simulink model "filecuaho"  (R2016b)
settings: Solver=VariableStepAuto  StartTime=0.0  StopTime=10.0  RelTol=1e-3
undefined symbols (not defined in the file): KACC_ACCT_CLR_NIDL_INIT, KACC_ACCUT_STATE_A, KACC_ACCUT_STATE_B, KACC_ACCUT_SW, KACC_ACTQSW, KACC_CLD, KACC_CLD_REQ_HYS, KACC_CLD_REQ_SW, KACC_COLPD, KACC_COMP_INRT, KACC_COMPTYPE_FIXED, KACC_COMPTYPE_VAR, KACC_CTTM_ACE, KACC_CTTM_ACON, KACC_CTTM_CRK, KACC_CTTM_FAN, KACC_CTTM_GRD, KACC_CTTM_IRS, KACC_CTTM_NAC, KACC_DIFFEVATEMPMAX, KACC_DIFFEVATEMPMIN, KACC_EVAT_ELSE, KACC_EVAT_ELSE_SW, KACC_EVATMPCUT_SW, KACC_EVATUPL_ELSE, KACC_EVATUPL_ELSE_SW, KACC_FANREQ_SW, KACC_FORCEDACON, KACC_HCAPS, KACC_HCAPS_HYS, KACC_HCCTTM, KACC_HCGRA, KACC_HCGRA_HYS, KACC_HCRGR, KACC_HCVS1, KACC_HCVS1_HYS, KACC_HCVS2, KACC_HCVS2_HYS, KACC_HEATUP_CE, KACC_HEATUP_CE_HYS, KACC_HEATUP_DRV2IDL, KACC_HEATUP_IDL2DRV, KACC_HEATUP_NE, KACC_HEATUP_NE_HYS, KACC_HIPS_ACOF, KACC_HIPS_ACON, KACC_LOPS_ACOF, KACC_LOPS_ACON, KACC_LYR3TR_ACHLD, KACC_NEW_RPM, KACC_OFDL_SW, KACC_OFDL_VCV, KACC_ONDL_SW, KACC_RECCP, KACC_RECCP_HYS, KACC_RECDLY, KACC_RECVS, KACC_S1_THWMAX, KACC_S1TM_THWULMT, KACC_SHLT_2CYL ... (+137)
libraries: lib2011b x727, SUBSYSTEM_LIB_CNV x30, SUBSYSTEM_LIB_ESC x2, SUBSYSTEM_LIB_AUX x1
(part 3 of 5)

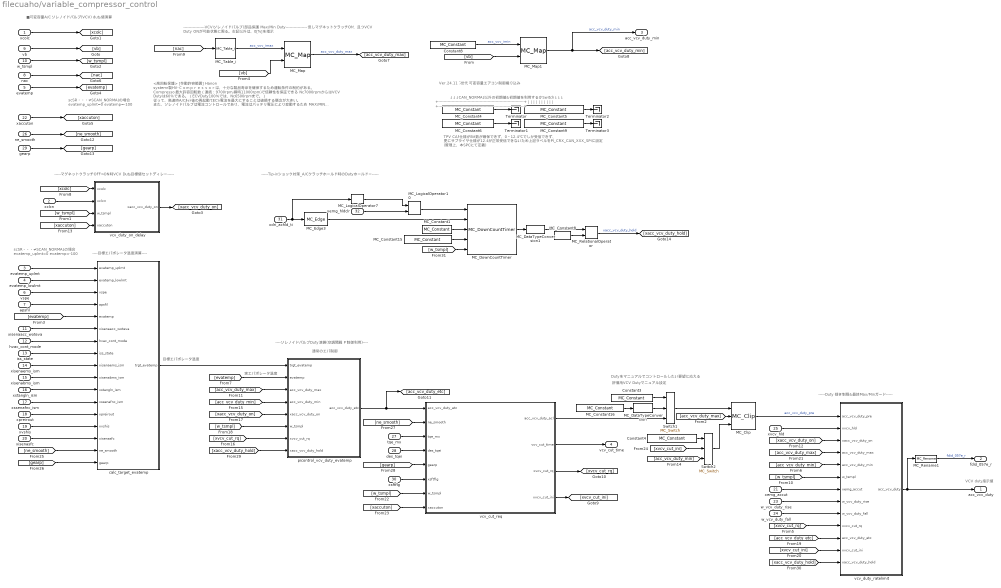
== system filecuaho/variable_compressor_control ==
  note: ■可変容量A/C ソレノイドバルブ(VCV) duty値演算
  note: VCV duty指示値
  note: <高回転保護>
      | [作動許容範囲]
      | Hanon systems製HV-Ｃｏｍｐｒｅｓｓｏｒは、十分な製品寿命を確保するため運転条件の制約がある。
      | Compressor最大許容回転数（連続：9700rpm/瞬時11000rpm)で信頼性を保証できる
      | Nc7000rpmからはVCV Dutyは60％である。（ECVDuty100％では、Nc6500rpmまで。）
      | 従って、高速時A/Cｶｯﾄ後の再起動でECV電流を最大にすることは破損する懸念が大きい。
      | また、ソレノイドバルブは電流コントロールであり、電流はバッテリ電圧により変動するため
      | MAX/MIN Dutyは電圧補正を行う
  note: 評価用VCV Dutyマニュアル設定
  note: Dutyをマニュアルでコントロールしたい要望に応える
  note: 通常のエバ制御
  note: 目標エバポレータ温度
  note: 実エバポレータ温度
  note: ----ソレノイドバルブDuty演算(空調開殿 PI制御利用)----
  note: scSR・・・≠SCAN_NORMALの場合
      |  evatemp_uplmt=0
      |  evatemp=-100
  note: ----目標エバポレータ温度演算----
  note: ----------------VCV(ソレノイドバルブ)部品保護 Max/Min Duty----------------
      | 但しマグネットクラッチON、且つVCV Duty ONが可能状態に限る。左記以外は、0[%]を指示
  note: scSR・・・≠SCAN_NORMALの場合
      |  evatemp_uplmt=0
      |  evatemp=-100
  note: -----マグネットクラッチOFF⇒ON時VCV Duty目標値セットディレー-----
  note: -----Duty 傾き制限&最終Max/Minガード-----
  note: ↓↓↓CAN_NORMAL以外の初期値&初期値を利用するかSwitch↓↓↓
  note: TPV CAN仕様がBit数が確保できず、0～12.4℃でしか受信できず、
      | 更にサプライヤ仕様が12.4が正常受信できないため上記ラベルをPI_CRX_CAN_XXX_SPCに設定
      | (管理上、本SPCにて定義)
  note: +----------------------------------------------------------------+
      | |                                                                                                                            　   |
      | |                                                                                                                            　   |
      | |                                                                                                                            　   |
      | |                                                                                                                            　   |
      | |                                                                                                                            　   |
      | +----------------------------------------------------------------+
  note: Ver.24.11
      | 7世代 可変容量エアコン制御織り込み
  note: -----Tip-inショック対策_A/Cクラッチホールド時のDutyホールドー-----
  xcolc : Inport
  xclcn : Inport  Port=2
  evatemp_uplmt : Inport  Port=3
  evatemp_lowlmt : Inport  Port=4
  evatemp : Inport  Port=5
  vspe : Inport  Port=6
  apsfil : Inport  Port=7
  nac : Inport  Port=8
  vb : Inport  Port=9
  w_tsmpl : Inport  Port=10
  xisenaacc_woteva : Inport  Port=11
  hvac_cont_mode : Inport  Port=12
  iss_state : Inport  Port=13
  xisenaems_ism : Inport  Port=14
  xisenabms_ism : Inport  Port=15
  xstangln_ism : Inport  Port=16
  xssenafnc_ism : Inport  Port=17
  xpreirout : Inport  Port=18
  xvshis : Inport  Port=19
  xisenasfc : Inport  Port=20
  xemg_accut : Inport  Port=21
  xaccuton : Inport  Port=22
  w_vcv_duty_rise : Inport  Port=23
  w_vcv_duty_fall : Inport  Port=24
  xvcv_hld : Inport  Port=25
  ne_smooth : Inport  Port=26
  tqe_mx : Inport  Port=27
  des_tqei : Inport  Port=28
  gearp : Inport  Port=29
  xsftflg : Inport  Port=30
  xdri_achld_ti : Inport  Port=31
  xemg_hldclr : Inport  Port=32
  Constant3 : lib2011b/Simulink Original/Sources/MC_Constant  Value=KACC_VCD_MN  datatype=Inherit: Inherit from 'Constant value'  SampleTime=inf  FramePeriod=inf  OutMin=[]  OutMax=[]  OutDataTypeStr=Inherit: Inherit from 'Constant value'
  Constant4 : lib2011b/Simulink Original/Sources/MC_Constant  Value=KACC_VCD_INIT  datatype=Inherit: Inherit from 'Constant value'  SampleTime=inf  FramePeriod=inf  OutMin=[]  OutMax=[]  OutDataTypeStr=Inherit: Inherit from 'Constant value'
  Constant8 : lib2011b/Simulink Original/Sources/MC_Constant  Value=KACC_VCD_IMIN  datatype=Inherit: Inherit from 'Constant value'  SampleTime=inf  FramePeriod=inf  OutMin=[]  OutMax=[]  OutDataTypeStr=Inherit: Inherit from 'Constant value'
  MC_Clip : lib2011b/Mazda Library/Other/MC_Clip
  MC_Constant1 : lib2011b/Simulink Original/Sources/MC_Constant  Value=true  datatype=Inherit: Inherit from 'Constant value'  SampleTime=inf  FramePeriod=inf  OutMin=[]  OutMax=[]  OutDataTypeStr=Inherit: Inherit from 'Constant value'
  MC_Constant15 : lib2011b/Simulink Original/Sources/MC_Constant  Value=KACC_SHLT_TIPIN  datatype=Inherit: Inherit from 'Constant value'  SampleTime=inf  FramePeriod=inf  OutMin=[]  OutMax=[]  OutDataTypeStr=Inherit: Inherit from 'Constant value'
  MC_Constant16 : lib2011b/Simulink Original/Sources/MC_Constant  Value=KACC_VCD_MNSW  datatype=Inherit: Inherit from 'Constant value'  SampleTime=inf  FramePeriod=inf  OutMin=[]  OutMax=[]  OutDataTypeStr=Inherit: Inherit from 'Constant value'
  MC_Constant4 : lib2011b/Simulink Original/Sources/MC_Constant  Value=KACC_EVAT_ELSE_SW  datatype=Inherit: Inherit from 'Constant value'  SampleTime=inf  FramePeriod=inf  OutMin=[]  OutMax=[]  OutDataTypeStr=Inherit: Inherit from 'Constant value'
  MC_Constant5 : lib2011b/Simulink Original/Sources/MC_Constant  Value=KACC_EVATUPL_ELSE_SW  datatype=Inherit: Inherit from 'Constant value'  SampleTime=inf  FramePeriod=inf  OutMin=[]  OutMax=[]  OutDataTypeStr=Inherit: Inherit from 'Constant value'
  MC_Constant6 : lib2011b/Simulink Original/Sources/MC_Constant  Value=KACC_EVAT_ELSE  datatype=Inherit: Inherit from 'Constant value'  SampleTime=inf  FramePeriod=inf  OutMin=[]  OutMax=[]  OutDataTypeStr=Inherit: Inherit from 'Constant value'
  MC_Constant8 : lib2011b/Simulink Original/Sources/MC_Constant  Value=0  datatype=uint16  SampleTime=inf  FramePeriod=inf  OutMin=[]  OutMax=[]  OutDataTypeStr=uint16
  MC_Constant9 : lib2011b/Simulink Original/Sources/MC_Constant  Value=KACC_EVATUPL_ELSE  datatype=Inherit: Inherit from 'Constant value'  SampleTime=inf  FramePeriod=inf  OutMin=[]  OutMax=[]  OutDataTypeStr=Inherit: Inherit from 'Constant value'
  MC_DataTypeConversion : lib2011b/Simulink Original/Signal Attributes/MC_DataTypeConversion  OutMin=[]  OutMax=[]  OutDataTypeStr=boolean  Signaltype=boolean  ConvertRealWorld=Real World Value (RWV)  RndMeth=Zero  SampleTime=-1
  MC_DataTypeConversion1 : lib2011b/Simulink Original/Signal Attributes/MC_DataTypeConversion  OutMin=[]  OutMax=[]  OutDataTypeStr=uint16  Signaltype=uint16  ConvertRealWorld=Real World Value (RWV)  RndMeth=Zero  SampleTime=-1
  MC_DownCountTimer : lib2011b/Mazda Library/Timer/MC_DownCountTimer
      settings: AttributesFormatString=DownCountTimer
  MC_Edge3 : lib2011b/Mazda Library/Other/MC_Edge
  MC_LogicalOperator10 : lib2011b/Simulink Original/Logic and Bit Operations/MC_LogicalOperator  SelectedOperator=OR  Inputs=2  SampleTime=-1  AllPortsSameDT=off  OutDataTypeStr=boolean
  MC_LogicalOperator7 : lib2011b/Simulink Original/Logic and Bit Operations/MC_LogicalOperator  SelectedOperator=NOT  Inputs=2  SampleTime=-1  AllPortsSameDT=off  OutDataTypeStr=boolean
  MC_Map : lib2011b/Simulink Original/Lookup Tables/MC_Map  Label=MACC_VCD_DUTY_VI  ColumnIndex=TACC_VCD_DUTY_VI_X  calsw_x=on  RowIndex=TACC_VCD_DUTY_VI_Y  calsw_y=on  OutputValues=MACC_VCD_DUTY_VI_Z
      settings: AttributesFormatString=%<Label>\nX-axis %<calsw_x>, Y-axis %<calsw_y>
  MC_Map1 : lib2011b/Simulink Original/Lookup Tables/MC_Map  Label=MACC_VCD_DUTY_VI  ColumnIndex=TACC_VCD_DUTY_VI_X  calsw_x=on  RowIndex=TACC_VCD_DUTY_VI_Y  calsw_y=on  OutputValues=MACC_VCD_DUTY_VI_Z
      settings: AttributesFormatString=%<Label>\nX-axis %<calsw_x>, Y-axis %<calsw_y>
  MC_RelationalOperator : lib2011b/Simulink Original/Logic and Bit Operations/MC_RelationalOperator  Operator=>  SampleTime=-1  InputSameDT=on  OutDataTypeStr=boolean
  MC_Rename1 : lib2011b/Mazda Library/Other/MC_Rename
  MC_Table_i : lib2011b/Simulink Original/Lookup Tables/MC_Table_i  Label=TACC_VCD_IMAX_NAC  InputValues=TACC_VCD_IMAX_NAC_X  calsw_x=on  OutputValues=TACC_VCD_IMAX_NAC_Y  LsbValue=LSB_TACC_VCD_IMAX_NAC_Y  OffsetValue=OFFSET_TACC_VCD_IMAX_NAC_Y
      settings: AttributesFormatString=%<Label>\nX-axis %<calsw_x>
  Switch1 : lib2011b/Simulink Original/Signal Routing/MC_Switch  Criteria=u2 ~= 0  Threshold=0  SampleTime=-1  InputSameDT=on  OutMin=[]  OutMax=[]  AllowDiffInputSizes=off
  Switch2 : lib2011b/Simulink Original/Signal Routing/MC_Switch  Criteria=u2 ~= 0  Threshold=0  SampleTime=-1  InputSameDT=on  OutMin=[]  OutMax=[]  AllowDiffInputSizes=off
  Terminator{,1..3} (4 alike) : Terminator
  calc_target_evatemp : Subsystem
  picontrol_vcv_duty_evatemp : Subsystem
  vcv_cut_req : Subsystem
      mask Display: disp('加速要求\n可変容量A/C指示Duty_OFF')
  vcv_duty_on_delay : Subsystem
  vcv_duty_ratelimit : Subsystem
  acc_vcv_duty : Outport
  fdid_057e_r : Outport  Port=2
  acc_vcv_duty_min : Outport  Port=3
  vcv_cut_time : Outport  Port=4
  wires:
  w_tsmpl/1 -> [w_tsmpl]
  evatemp/1 -> [evatemp]
  evatemp_uplmt/1 -> calc_target_evatemp/1(evatemp_uplmt)
  MC_DataTypeConversion/1 -> Switch1/2
  MC_Constant16/1 -> MC_DataTypeConversion/1
  nac/1 -> [nac]
  [nac] -> MC_Table_i/1
  [vb] -> MC_Map/2
  MC_Map/1 -> [acc_vcv_duty_max]  "acc_vcv_duty_max"
  [acc_vcv_duty_max] -> MC_Clip/2
  MC_Map1/1 -> [acc_vcv_duty_min], acc_vcv_duty_min/1  "acc_vcv_duty_min"
  calc_target_evatemp/1(trgt_evatemp) -> picontrol_vcv_duty_evatemp/1(trgt_evatemp)
  vspe/1 -> calc_target_evatemp/3(vspe)
  [w_tsmpl] -> vcv_duty_on_delay/3(w_tsmpl)
  Constant3/1 -> Switch1/1
  apsfil/1 -> calc_target_evatemp/4(apsfil)
  evatemp_lowlmt/1 -> calc_target_evatemp/2(evatemp_lowlmt)
  [evatemp] -> calc_target_evatemp/5(evatemp)
  MC_Table_i/1 -> MC_Map/1  "acc_vcv_imax"
  Constant8/1 -> MC_Map1/1  "acc_vcv_imin"
  vb/1 -> [vb]
  [vb] -> MC_Map1/2
  [xcolc] -> vcv_duty_on_delay/1(xcolc)
  xcolc/1 -> [xcolc]
  vcv_duty_on_delay/1(xacc_vcv_duty_on) -> [xacc_vcv_duty_on]
  Switch1/1 -> MC_Clip/1
  xclcn/1 -> vcv_duty_on_delay/2(xclcn)
  MC_Constant4/1 -> Terminator/1
  MC_Constant6/1 -> Terminator1/1
  MC_Constant5/1 -> Terminator2/1
  MC_Constant9/1 -> Terminator3/1
  xisenaacc_woteva/1 -> calc_target_evatemp/6(xisenaacc_woteva)
  hvac_cont_mode/1 -> calc_target_evatemp/7(hvac_cont_mode)
  iss_state/1 -> calc_target_evatemp/8(iss_state)
  xisenaems_ism/1 -> calc_target_evatemp/9(xisenaems_ism)
  xisenabms_ism/1 -> calc_target_evatemp/10(xisenabms_ism)
  xstangln_ism/1 -> calc_target_evatemp/11(xstangln_ism)
  xssenafnc_ism/1 -> calc_target_evatemp/12(xssenafnc_ism)
  xpreirout/1 -> calc_target_evatemp/13(xpreirout)
  xvshis/1 -> calc_target_evatemp/14(xvshis)
  xisenasfc/1 -> calc_target_evatemp/15(xisenasfc)
  MC_Rename1/1 -> fdid_057e_r/1  "fdid_057e_r"
  [evatemp] -> picontrol_vcv_duty_evatemp/2(evatemp)
  [acc_vcv_duty_max] -> picontrol_vcv_duty_evatemp/3(acc_vcv_duty_max)
  [acc_vcv_duty_min] -> picontrol_vcv_duty_evatemp/4(acc_vcv_duty_min)
  [xacc_vcv_duty_on] -> picontrol_vcv_duty_evatemp/5(xacc_vcv_duty_on)
  [w_tsmpl] -> picontrol_vcv_duty_evatemp/6(w_tsmpl)
  picontrol_vcv_duty_evatemp/1(acc_vcv_duty_etc) -> vcv_cut_req/1(acc_vcv_duty_etc), [acc_vcv_duty_etc]
  vcv_cut_req/1(acc_vcv_duty_acl) -> Switch1/3
  xaccuton/1 -> [xaccuton]
  [xaccuton] -> vcv_duty_on_delay/4(xaccuton)
  Constant4/1 -> Switch2/1
  [xvcv_cut_ini] -> Switch2/2
  [acc_vcv_duty_min] -> Switch2/3
  Switch2/1 -> MC_Clip/3
  tqe_mx/1 -> vcv_cut_req/3(tqe_mx)
  des_tqei/1 -> vcv_cut_req/4(des_tqei)
  xsftflg/1 -> vcv_cut_req/6(xsftflg)
  [w_tsmpl] -> vcv_cut_req/7(w_tsmpl)
  [xaccuton] -> vcv_cut_req/8(xaccuton)
  vcv_cut_req/2(vcv_cut_time) -> vcv_cut_time/1
  vcv_duty_ratelimit/1(acc_vcv_duty) -> acc_vcv_duty/1, MC_Rename1/1
  [xvcv_cut_rq] -> picontrol_vcv_duty_evatemp/7(xvcv_cut_rq)
  vcv_cut_req/3(xvcv_cut_rq) -> [xvcv_cut_rq]
  vcv_cut_req/4(xvcv_cut_ini) -> [xvcv_cut_ini]
  MC_Clip/1 -> vcv_duty_ratelimit/1(acc_vcv_duty_pre)  "acc_vcv_duty_pre"
  xvcv_hld/1 -> vcv_duty_ratelimit/2(xvcv_hld)
  [xacc_vcv_duty_on] -> vcv_duty_ratelimit/3(xacc_vcv_duty_on)
  [acc_vcv_duty_max] -> vcv_duty_ratelimit/4(acc_vcv_duty_max)
  [acc_vcv_duty_min] -> vcv_duty_ratelimit/5(acc_vcv_duty_min)
  [w_tsmpl] -> vcv_duty_ratelimit/6(w_tsmpl)
  xemg_accut/1 -> vcv_duty_ratelimit/7(xemg_accut)
  w_vcv_duty_rise/1 -> vcv_duty_ratelimit/8(w_vcv_duty_rise)
  w_vcv_duty_fall/1 -> vcv_duty_ratelimit/9(w_vcv_duty_fall)
  [xvcv_cut_rq] -> vcv_duty_ratelimit/10(xvcv_cut_rq)
  [acc_vcv_duty_etc] -> vcv_duty_ratelimit/11(acc_vcv_duty_etc)
  [xvcv_cut_ini] -> vcv_duty_ratelimit/12(xvcv_cut_ini)
  [ne_smooth] -> calc_target_evatemp/16(ne_smooth)
  [gearp] -> calc_target_evatemp/17(gearp)
  [ne_smooth] -> vcv_cut_req/2(ne_smooth)
  [gearp] -> vcv_cut_req/5(gearp)
  ne_smooth/1 -> [ne_smooth]
  gearp/1 -> [gearp]
  [xacc_vcv_duty_hold] -> picontrol_vcv_duty_evatemp/8(xacc_vcv_duty_hold)
  [xacc_vcv_duty_hold] -> vcv_duty_ratelimit/13(xacc_vcv_duty_hold)
  MC_Constant8/1 -> MC_RelationalOperator/2
  MC_Constant1/1 -> MC_DownCountTimer/3
  [w_tsmpl] -> MC_DownCountTimer/5
  MC_LogicalOperator7/1 -> MC_LogicalOperator10/1
  xemg_hldclr/1 -> MC_LogicalOperator10/2
  MC_LogicalOperator10/1 -> MC_DownCountTimer/1
  MC_DownCountTimer/1 -> MC_DataTypeConversion1/1
  MC_DataTypeConversion1/1 -> MC_RelationalOperator/1
  MC_Constant15/1 -> MC_DownCountTimer/4
  MC_Edge3/1 -> MC_DownCountTimer/2
  MC_RelationalOperator/1 -> [xacc_vcv_duty_hold]  "xacc_vcv_duty_hold"
  xdri_achld_ti/1 -> MC_Edge3/1, MC_LogicalOperator7/1

== system filecuaho/acc_control/vcv_duty_hold_time ==
  note: TXVがシャットオフ⇔オンによるDutyハンチングを
      | 防止するため冷媒圧が低い場合は傾き制限を
      | 有効とする。
  colp : Inport
  w_tsmpl : Inport  Port=2
  acc_vcv_duty : Inport  Port=3
  w_acc_vcv_duty_min : Inport  Port=4
  xaccuton : Inport  Port=5
  Constant1 : lib2011b/Simulink Original/Sources/MC_Constant  Value=KACC_VCD_RLMT_COLP  datatype=Inherit: Inherit from 'Constant value'  SampleTime=inf  FramePeriod=inf  OutMin=[]  OutMax=[]  OutDataTypeStr=Inherit: Inherit from 'Constant value'
  Constant11 : lib2011b/Simulink Original/Sources/MC_Constant  Value=KACC_VCD_RLMTF  datatype=Inherit: Inherit from 'Constant value'  SampleTime=inf  FramePeriod=inf  OutMin=[]  OutMax=[]  OutDataTypeStr=Inherit: Inherit from 'Constant value'
  Constant12 : lib2011b/Simulink Original/Sources/MC_Constant  Value=KACC_VCD_RLMTR_COLP  datatype=Inherit: Inherit from 'Constant value'  SampleTime=inf  FramePeriod=inf  OutMin=[]  OutMax=[]  OutDataTypeStr=Inherit: Inherit from 'Constant value'
  Constant13 : lib2011b/Simulink Original/Sources/MC_Constant  Value=KACC_VCD_RLMTF_COLP  datatype=Inherit: Inherit from 'Constant value'  SampleTime=inf  FramePeriod=inf  OutMin=[]  OutMax=[]  OutDataTypeStr=Inherit: Inherit from 'Constant value'
  Constant3 : lib2011b/Simulink Original/Sources/MC_Constant  Value=KACC_VCD_HOLD  datatype=Inherit: Inherit from 'Constant value'  SampleTime=inf  FramePeriod=inf  OutMin=[]  OutMax=[]  OutDataTypeStr=Inherit: Inherit from 'Constant value'
  Constant9 : lib2011b/Simulink Original/Sources/MC_Constant  Value=KACC_VCD_RLMTR  datatype=Inherit: Inherit from 'Constant value'  SampleTime=inf  FramePeriod=inf  OutMin=[]  OutMax=[]  OutDataTypeStr=Inherit: Inherit from 'Constant value'
  MC_Abs1 : lib2011b/Simulink Original/Math Operations/MC_Abs  SampleTime=-1  OutMin=[]  OutMax=[]  OutDataTypeStr=single
  MC_Add : lib2011b/Simulink Original/Math Operations/MC_Add  Inputs=++  CollapseDim=1  SampleTime=-1  InputSameDT=on  OutMin=[]  OutMax=[]  OutDataTypeStr=single
  MC_Add1 : lib2011b/Simulink Original/Math Operations/MC_Add  Inputs=+-  CollapseDim=1  SampleTime=-1  InputSameDT=on  OutMin=[]  OutMax=[]  OutDataTypeStr=single
  MC_Div_ZERO : lib2011b/Mazda Library/Other/MC_Div_ZERO  threshold=1e-10  threshold_bg=1e-10
      settings: AttributesFormatString=Threshold=%<threshold>
  MC_LogicalOperator4 : lib2011b/Simulink Original/Logic and Bit Operations/MC_LogicalOperator  SelectedOperator=AND  Inputs=2  SampleTime=-1  AllPortsSameDT=off  OutDataTypeStr=boolean
  MC_RelationalOperator1 : lib2011b/Simulink Original/Logic and Bit Operations/MC_RelationalOperator  Operator=>  SampleTime=-1  InputSameDT=on  OutDataTypeStr=boolean
  MC_RelationalOperator2 : lib2011b/Simulink Original/Logic and Bit Operations/MC_RelationalOperator  Operator=<  SampleTime=-1  InputSameDT=on  OutDataTypeStr=boolean
  Switch5 : lib2011b/Simulink Original/Signal Routing/MC_Switch  Criteria=u2 ~= 0  Threshold=0  SampleTime=-1  InputSameDT=on  OutMin=[]  OutMax=[]  AllowDiffInputSizes=off
  Switch6 : lib2011b/Simulink Original/Signal Routing/MC_Switch  Criteria=u2 ~= 0  Threshold=0  SampleTime=-1  InputSameDT=on  OutMin=[]  OutMax=[]  AllowDiffInputSizes=off
  w_vcv_duty_rise : Outport
  w_vcv_duty_fall : Outport  Port=2
  xvcv_hld : Outport  Port=3
  w_vcv_hld_time : Outport  Port=4
  wires:
  colp/1 -> MC_RelationalOperator2/1
  Constant1/1 -> MC_RelationalOperator2/2
  Constant13/1 -> Switch5/1
  MC_RelationalOperator2/1 -> Switch6/2, Switch5/2
  Constant12/1 -> Switch6/1
  Constant11/1 -> Switch5/3
  Constant9/1 -> Switch6/3
  Switch6/1 -> w_vcv_duty_rise/1  "w_vcv_duty_rise"
  Switch5/1 -> w_vcv_duty_fall/1, MC_Abs1/1  "w_vcv_duty_fall"
  Constant3/1 -> MC_Add/2
  acc_vcv_duty/1 -> MC_RelationalOperator1/1, MC_Div_ZERO/1
  MC_Add/1 -> MC_RelationalOperator1/2
  MC_RelationalOperator1/1 -> MC_LogicalOperator4/1
  MC_Abs1/1 -> MC_Div_ZERO/2
  MC_Div_ZERO/1 -> MC_Add1/1
  w_tsmpl/1 -> MC_Add1/2
  MC_LogicalOperator4/1 -> xvcv_hld/1  "xvcv_hld"
  MC_Add1/1 -> w_vcv_hld_time/1  "w_vcv_hld_time"
  xaccuton/1 -> MC_LogicalOperator4/2
  w_acc_vcv_duty_min/1 -> MC_Add/1

== system filecuaho/acc_tqe/AC_reserve_tq ==
  ac_ppm_tmr : Inport
  xcolc : Inport  Port=2
  trans_peak_time : Inport  Port=3
  trans_peak_actq : Inport  Port=4
  tqe_trans_ac : Inport  Port=5
  MC_Add : lib2011b/Simulink Original/Math Operations/MC_Add  Inputs=++  CollapseDim=1  SampleTime=-1  InputSameDT=on  OutMin=[]  OutMax=[]  OutDataTypeStr=single
  MC_Constant1 : lib2011b/Simulink Original/Sources/MC_Constant  Value=0  datatype=single  SampleTime=inf  FramePeriod=inf  OutMin=[]  OutMax=[]  OutDataTypeStr=single
  MC_Constant2 : lib2011b/Simulink Original/Sources/MC_Constant  Value=KACC_ACTQSW  datatype=Inherit: Inherit from 'Constant value'  SampleTime=inf  FramePeriod=inf  OutMin=[]  OutMax=[]  OutDataTypeStr=Inherit: Inherit from 'Constant value'
  MC_DataTypeConversion : lib2011b/Simulink Original/Signal Attributes/MC_DataTypeConversion  OutMin=[]  OutMax=[]  OutDataTypeStr=boolean  Signaltype=boolean  ConvertRealWorld=Real World Value (RWV)  RndMeth=Zero  SampleTime=-1
  MC_LogicalOperator1 : lib2011b/Simulink Original/Logic and Bit Operations/MC_LogicalOperator  SelectedOperator=AND  Inputs=3  SampleTime=-1  AllPortsSameDT=off  OutDataTypeStr=boolean
  MC_RelationalOperator : lib2011b/Simulink Original/Logic and Bit Operations/MC_RelationalOperator  Operator=<  SampleTime=-1  InputSameDT=on  OutDataTypeStr=boolean
  MC_Switch1 : lib2011b/Simulink Original/Signal Routing/MC_Switch  Criteria=u2 ~= 0  Threshold=0  SampleTime=-1  InputSameDT=on  OutMin=[]  OutMax=[]  AllowDiffInputSizes=off
  w_tqe_rsv_ac_old : Outport
  wires:
  trans_peak_time/1 -> [trans_peak_time]
  trans_peak_actq/1 -> [trans_peak_actq]
  tqe_trans_ac/1 -> [tqe_trans_ac]
  ac_ppm_tmr/1 -> [ac_ppm_tmr]
  xcolc/1 -> [xcolc]
  [trans_peak_actq] -> MC_Add/1
  [tqe_trans_ac] -> MC_Add/2
  [ac_ppm_tmr] -> MC_RelationalOperator/1
  [trans_peak_time] -> MC_RelationalOperator/2
  [xcolc] -> MC_LogicalOperator1/2
  MC_LogicalOperator1/1 -> MC_Switch1/2  "xrsvtqe_ac"
  MC_Constant1/1 -> MC_Switch1/3
  MC_Constant2/1 -> MC_DataTypeConversion/1
  MC_DataTypeConversion/1 -> MC_LogicalOperator1/3
  MC_RelationalOperator/1 -> MC_LogicalOperator1/1
  MC_Switch1/1 -> w_tqe_rsv_ac_old/1  "w_tqe_rsv_ac_old"
  MC_Add/1 -> MC_Switch1/1

== system filecuaho/acc_tqe/AC_reserve_tq_new ==
  note: (-)
  note: (+)
  note: (+)
  note: "余裕トルク"="クラッチ締結後トルク(推定値)"-"現トルク"
      | ※負荷トルクは負値であることに注意
      |
      | [コメント]
      |  クラッチ締結後現トルクが挙がってくると上記引き算により
      |  徐々にリザーブが絞られる
  note: クラッチ締結後トルク
  note: inertia以外
  note: inertia
  note: クラッチに依らず常時算出
  tqe_ac_new : Inport
  tqe_ac_inrt_rsv : Inport  Port=2
  tqe_ac_rsv_new : Inport  Port=3
  xcolc : Inport  Port=4
  xclcn : Inport  Port=5
  MC_Add1 : lib2011b/Simulink Original/Math Operations/MC_Add  Inputs=++  CollapseDim=1  SampleTime=-1  InputSameDT=on  OutMin=[]  OutMax=[]  OutDataTypeStr=single
  MC_Add2 : lib2011b/Simulink Original/Math Operations/MC_Add  Inputs=++  CollapseDim=1  SampleTime=-1  InputSameDT=on  OutMin=[]  OutMax=[]  OutDataTypeStr=single
  MC_Constant1 : lib2011b/Simulink Original/Sources/MC_Constant  Value=KACC_TQERSV_SW  datatype=Inherit: Inherit from 'Constant value'  SampleTime=inf  FramePeriod=inf  OutMin=[]  OutMax=[]  OutDataTypeStr=Inherit: Inherit from 'Constant value'
  MC_Constant6 : lib2011b/Simulink Original/Sources/MC_Constant  Value=0  datatype=single  SampleTime=inf  FramePeriod=inf  OutMin=[]  OutMax=[]  OutDataTypeStr=single
  MC_DataTypeConversion : lib2011b/Simulink Original/Signal Attributes/MC_DataTypeConversion  OutMin=[]  OutMax=[]  OutDataTypeStr=boolean  Signaltype=boolean  ConvertRealWorld=Real World Value (RWV)  RndMeth=Zero  SampleTime=-1
  MC_LogicalOperator1 : lib2011b/Simulink Original/Logic and Bit Operations/MC_LogicalOperator  SelectedOperator=AND  Inputs=2  SampleTime=-1  AllPortsSameDT=off  OutDataTypeStr=boolean
  MC_LogicalOperator2 : lib2011b/Simulink Original/Logic and Bit Operations/MC_LogicalOperator  SelectedOperator=OR  Inputs=2  SampleTime=-1  AllPortsSameDT=off  OutDataTypeStr=boolean
  MC_Switch5 : lib2011b/Simulink Original/Signal Routing/MC_Switch  Criteria=u2 ~= 0  Threshold=0  SampleTime=-1  InputSameDT=on  OutMin=[]  OutMax=[]  AllowDiffInputSizes=off
  tqe_rsv_ac_new : Outport
  wires:
  tqe_ac_inrt_rsv/1 -> MC_Add1/1
  tqe_ac_rsv_new/1 -> MC_Add1/2
  tqe_ac_new/1 -> MC_Add2/1
  MC_Add2/1 -> MC_Switch5/1
  xclcn/1 -> MC_LogicalOperator2/2
  MC_Constant6/1 -> MC_Switch5/3
  MC_Add1/1 -> MC_Add2/2
  xcolc/1 -> MC_LogicalOperator2/1
  MC_Switch5/1 -> tqe_rsv_ac_new/1  "tqe_rsv_ac_new"
  MC_Constant1/1 -> MC_DataTypeConversion/1
  MC_LogicalOperator2/1 -> MC_LogicalOperator1/1
  MC_DataTypeConversion/1 -> MC_LogicalOperator1/2
  MC_LogicalOperator1/1 -> MC_Switch5/2

== system filecuaho/acc_tqe/AC_rush_tq ==
  note: /* A/Cプーリー比 */
  note: /* 負荷TQを正で出力 */
  note: /* 負荷TQを負で出力 */
  note: /* 過渡時でもクラッチOFFで負荷は"0" */
  note: /* エンジン負荷TQは負値で出力 */
  note: /* 過渡負荷（ラッシュTQ）をPEAK時間とPEAK負荷から2次関数で表現する */
  note: /* A/Cプーリー比 */
  ac_ppm_tmr : Inport
  ne_pred_tqm : Inport  Port=2
  colp : Inport  Port=3
  xcolc : Inport  Port=4
  MC_Add : lib2011b/Simulink Original/Math Operations/MC_Add  Inputs=+-  CollapseDim=1  SampleTime=-1  InputSameDT=on  OutMin=[]  OutMax=[]  OutDataTypeStr=single
  MC_Constant : lib2011b/Simulink Original/Sources/MC_Constant  Value=KACPULY  datatype=Inherit: Inherit from 'Constant value'  SampleTime=inf  FramePeriod=inf  OutMin=[]  OutMax=[]  OutDataTypeStr=Inherit: Inherit from 'Constant value'
  MC_Constant1 : lib2011b/Simulink Original/Sources/MC_Constant  Value=0  datatype=single  SampleTime=inf  FramePeriod=inf  OutMin=[]  OutMax=[]  OutDataTypeStr=single
  MC_Constant2 : lib2011b/Simulink Original/Sources/MC_Constant  Value=-1  datatype=single  SampleTime=inf  FramePeriod=inf  OutMin=[]  OutMax=[]  OutDataTypeStr=single
  MC_Constant3 : lib2011b/Simulink Original/Sources/MC_Constant  Value=2  datatype=single  SampleTime=inf  FramePeriod=inf  OutMin=[]  OutMax=[]  OutDataTypeStr=single
  MC_Constant4 : lib2011b/Simulink Original/Sources/MC_Constant  Value=-1  datatype=single  SampleTime=inf  FramePeriod=inf  OutMin=[]  OutMax=[]  OutDataTypeStr=single
  MC_Constant5 : lib2011b/Simulink Original/Sources/MC_Constant  Value=0  datatype=single  SampleTime=inf  FramePeriod=inf  OutMin=[]  OutMax=[]  OutDataTypeStr=single
  MC_Constant6 : lib2011b/Simulink Original/Sources/MC_Constant  Value=KACPULY  datatype=Inherit: Inherit from 'Constant value'  SampleTime=inf  FramePeriod=inf  OutMin=[]  OutMax=[]  OutDataTypeStr=Inherit: Inherit from 'Constant value'
  MC_Constant7 : lib2011b/Simulink Original/Sources/MC_Constant  Value=0  datatype=single  SampleTime=inf  FramePeriod=inf  OutMin=[]  OutMax=[]  OutDataTypeStr=single
  MC_Map : lib2011b/Simulink Original/Lookup Tables/MC_Map_i  Label=MACC_PEAKACTQ  ColumnIndex=TACC_PEAKACTQ_X  calsw_x=on  RowIndex=TACC_PEAKACTQ_Y  calsw_y=on  OutputValues=MACC_PEAKACTQ_Z  LsbValue=LSB_MACC_PEAKACTQ_Z  OffsetValue=OFFSET_MACC_PEAKACTQ_Z
      settings: AttributesFormatString=%<Label>\nX-axis %<calsw_x>, Y-axis %<calsw_y>
  MC_Map1 : lib2011b/Simulink Original/Lookup Tables/MC_Map_i  Label=MACC_PEAKTIME  ColumnIndex=TACC_PEAKTIME_X  calsw_x=on  RowIndex=TACC_PEAKTIME_Y  calsw_y=on  OutputValues=MACC_PEAKTIME_Z  LsbValue=LSB_MACC_PEAKTIME_Z  OffsetValue=OFFSET_MACC_PEAKTIME_Z
      settings: AttributesFormatString=%<Label>\nX-axis %<calsw_x>, Y-axis %<calsw_y>
  MC_MinMax : lib2011b/Simulink Original/Math Operations/MC_MinMax  Function=min  Inputs=2  SampleTime=-1  InputSameDT=on  OutMin=[]  OutMax=[]
  MC_Product{1..2,4,6} (4 alike) : lib2011b/Simulink Original/Math Operations/MC_Product  Inputs=**  Multiplication=Element-wise(.*)  CollapseDim=1  SampleTime=-1  OutMin=[]  OutMax=[]  OutDataTypeStr=single  RndMeth=Zero
  MC_Product3 : lib2011b/Simulink Original/Math Operations/MC_Product  Inputs=***  Multiplication=Element-wise(.*)  CollapseDim=1  SampleTime=-1  OutMin=[]  OutMax=[]  OutDataTypeStr=single  RndMeth=Zero
  MC_Product5 : lib2011b/Simulink Original/Math Operations/MC_Product  Inputs=**//  Multiplication=Element-wise(.*)  CollapseDim=1  SampleTime=-1  OutMin=[]  OutMax=[]  OutDataTypeStr=single  RndMeth=Zero
  MC_RelationalOperator : lib2011b/Simulink Original/Logic and Bit Operations/MC_RelationalOperator  Operator=>  SampleTime=-1  InputSameDT=on  OutDataTypeStr=boolean
  MC_Switch : lib2011b/Simulink Original/Signal Routing/MC_Switch  Criteria=u2 ~= 0  Threshold=0  SampleTime=-1  InputSameDT=on  OutMin=[]  OutMax=[]  AllowDiffInputSizes=off
  MC_Switch1 : lib2011b/Simulink Original/Signal Routing/MC_Switch  Criteria=u2 ~= 0  Threshold=0  SampleTime=-1  InputSameDT=on  OutMin=[]  OutMax=[]  AllowDiffInputSizes=off
  MC_Switch2 : lib2011b/Simulink Original/Signal Routing/MC_Switch  Criteria=u2 ~= 0  Threshold=0  SampleTime=-1  InputSameDT=on  OutMin=[]  OutMax=[]  AllowDiffInputSizes=off
  MC_UnitDelay : lib2011b/Simulink Original/Discrete/MC_UnitDelay  InitialCondition=0  InputProcessing=Inherited  SampleTime=-1  StateName=delay_yclcn_b20m9493
      settings: StateMustResolveToSignalObject=off  StateStorageClass=ExportedGlobal
  MC_UnitDelay1 : lib2011b/Simulink Original/Discrete/MC_UnitDelay  InitialCondition=0  InputProcessing=Inherited  SampleTime=-1  StateName=delay_yclcn_b20m9494
      settings: StateMustResolveToSignalObject=off  StateStorageClass=ExportedGlobal
  tqe_trans_ac : Outport
  trans_peak_actq : Outport  Port=2
  trans_peak_time : Outport  Port=3
  nac : Outport  Port=4
  wires:
  MC_Product1/1 -> MC_Switch/3, nac/1  "nac"
  ne_pred_tqm/1 -> MC_Product1/1
  MC_Constant/1 -> MC_Product1/2
  colp/1 -> MC_Switch1/3
  MC_UnitDelay1/1 -> MC_Switch1/1
  MC_UnitDelay/1 -> MC_Switch/1
  MC_Switch/1 -> MC_UnitDelay/1, [rush_cor_nac]  "rush_cor_nac"
  MC_Switch1/1 -> MC_UnitDelay1/1, [rush_cor_colp]  "rush_cor_colp"
  xcolc/1 -> [xcolc]
  [xcolc] -> MC_Switch/2
  [xcolc] -> MC_Switch1/2
  MC_Constant1/1 -> MC_MinMax/2
  MC_Product2/1 -> MC_MinMax/1
  MC_Constant2/1 -> MC_Product2/2
  ac_ppm_tmr/1 -> [ac_ppm_tmr]
  [rush_cor_colp] -> MC_Map/1
  [rush_cor_nac] -> MC_Map/2
  [rush_cor_colp] -> MC_Map1/1
  [rush_cor_nac] -> MC_Map1/2
  MC_Map1/1 -> [trans_peak_time]  "trans_peak_time"
  MC_Product3/1 -> MC_Product2/1
  MC_Add/1 -> MC_Product3/3
  [ac_ppm_tmr] -> MC_Product3/2, MC_Add/1
  MC_Product4/1 -> MC_Add/2
  MC_Constant3/1 -> MC_Product4/1
  [trans_peak_time] -> MC_Product4/2
  MC_Product5/1 -> MC_Product3/1
  MC_Constant4/1 -> MC_Product5/1
  [trans_peak_actq] -> MC_Product5/2
  [trans_peak_time] -> MC_Product5/3, MC_Product5/4
  [trans_peak_actq] -> trans_peak_actq/1
  [trans_peak_time] -> trans_peak_time/1
  MC_MinMax/1 -> MC_Switch2/1
  MC_Switch2/1 -> tqe_trans_ac/1  "tqe_trans_ac"
  MC_Constant5/1 -> MC_Switch2/3
  MC_Map/1 -> MC_Product6/1
  MC_Product6/1 -> [trans_peak_actq]  "trans_peak_actq"
  MC_Constant6/1 -> MC_Product6/2
  [ac_ppm_tmr] -> MC_RelationalOperator/1
  MC_RelationalOperator/1 -> MC_Switch2/2
  MC_Constant7/1 -> MC_RelationalOperator/2

== system filecuaho/acc_tqe/ac_inertia_torque ==
  note: ロストルク（信号)は
      | 負であらわす
  note: A/Cプーリー比
  note: 可変容量コンプレッサトルク推定(イナーシャトルク算出)
  note: nac:マグネットクラッチON/OFFによらずエンジン回転数×プーリー比で算出
  note: /* マグネットクラッチON時のイナーシャ成分演算 */
  note: /* 冷媒圧によるエアコン負荷演算 (R134a用)*/
  note: マグネットクラッチON/OFFディレーを掛ける前の指示
  note: マグネットクラッチON/OFFディレーを掛けた後の指示
  note: リザーブ用であるため
      | 負値⇒正値に変更
  note: (+)
  note: (-)
  nac : Inport
  xclcn : Inport  Port=2
  xcolc : Inport  Port=3
  clacdl : Inport  Port=4
  w_tsmpl : Inport  Port=5
  ne_pred_tqm : Inport  Port=6
  Constant1 : lib2011b/Simulink Original/Sources/MC_Constant  Value=-1  datatype=single  SampleTime=inf  FramePeriod=inf  OutMin=[]  OutMax=[]  OutDataTypeStr=single
  Constant4 : lib2011b/Simulink Original/Sources/MC_Constant  Value=-1  datatype=single  SampleTime=inf  FramePeriod=inf  OutMin=[]  OutMax=[]  OutDataTypeStr=single
  MC_Constant : lib2011b/Simulink Original/Sources/MC_Constant  Value=KACPULY  datatype=Inherit: Inherit from 'Constant value'  SampleTime=inf  FramePeriod=inf  OutMin=[]  OutMax=[]  OutDataTypeStr=Inherit: Inherit from 'Constant value'
  MC_Constant7 : lib2011b/Simulink Original/Sources/MC_Constant  Value=0  datatype=single  SampleTime=inf  FramePeriod=inf  OutMin=[]  OutMax=[]  OutDataTypeStr=single
  MC_Product2 : lib2011b/Simulink Original/Math Operations/MC_Product  Inputs=***  Multiplication=Element-wise(.*)  CollapseDim=1  SampleTime=-1  OutMin=[]  OutMax=[]  OutDataTypeStr=single  RndMeth=Zero
  MC_Switch4 : lib2011b/Simulink Original/Signal Routing/MC_Switch  Criteria=u2 ~= 0  Threshold=0  SampleTime=-1  InputSameDT=on  OutMin=[]  OutMax=[]  AllowDiffInputSizes=off
  MC_Table : lib2011b/Simulink Original/Lookup Tables/MC_Table  Label=TACC_INRT_GAIN  InputValues=TACC_INRT_GAIN_X  calsw_x=on  OutputValues=TACC_INRT_GAIN_Y
      settings: AttributesFormatString=%<Label>\nX-axis %<calsw_x>
  Product1 : lib2011b/Simulink Original/Math Operations/MC_Product  Inputs=**  Multiplication=Element-wise(.*)  CollapseDim=1  SampleTime=-1  OutMin=[]  OutMax=[]  OutDataTypeStr=single  RndMeth=Zero
  Product2 : lib2011b/Simulink Original/Math Operations/MC_Product  Inputs=**  Multiplication=Element-wise(.*)  CollapseDim=1  SampleTime=-1  OutMin=[]  OutMax=[]  OutDataTypeStr=single  RndMeth=Zero
  ac_torque_estimation_inrtia : Subsystem
  tqe_ac_inrt : Outport
  tqe_ac_inrt_rsv : Outport  Port=2
  wires:
  nac/1 -> ac_torque_estimation_inrtia/1(nac)
  xcolc/1 -> [xcolc]
  xclcn/1 -> [xclcn]
  [xcolc] -> ac_torque_estimation_inrtia/2(xcolc)
  clacdl/1 -> ac_torque_estimation_inrtia/3(clacdl)
  w_tsmpl/1 -> ac_torque_estimation_inrtia/4(w_tsmpl)
  Constant1/1 -> MC_Product2/1
  MC_Constant/1 -> MC_Product2/2
  ac_torque_estimation_inrtia/1(tqac_new_inrt) -> MC_Product2/3
  MC_Constant7/1 -> MC_Switch4/3
  [xclcn] -> MC_Switch4/2
  MC_Switch4/1 -> tqe_ac_inrt/1  "tqe_ac_inrt"
  Constant4/1 -> Product1/1
  Product1/1 -> tqe_ac_inrt_rsv/1  "tqe_ac_inrt_rsv"
  MC_Product2/1 -> Product2/1
  Product2/1 -> MC_Switch4/1, Product1/2
  MC_Table/1 -> Product2/2
  ne_pred_tqm/1 -> MC_Table/1

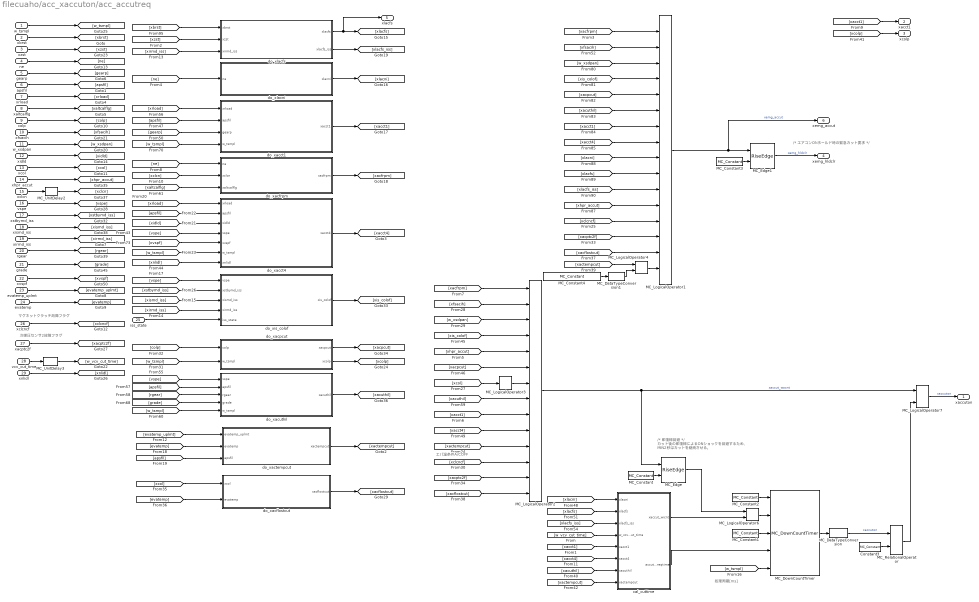
== system filecuaho/acc_xaccuton/acc_accutreq ==
  note: /* 即復帰回避 */
      | カット後の即復帰によるONショックを回避するため、
      | MIN2秒はカットを継続させる。
  note: /* エアコンONホールド時の緊急カット要求 */
  note: 処理周期[ms]
  note: エバ温条件A/COFF
  note: マグネットクラッチ故障フラグ
  note: 冷媒圧センサ2故障フラグ
  w_tsmpl : Inport
  xbrst : Inport  Port=2
  xzst : Inport  Port=3
  ne : Inport  Port=4
  gearp : Inport  Port=5
  apsfil : Inport  Port=6
  xrload : Inport  Port=7
  xaltcalflg : Inport  Port=8
  colp : Inport  Port=9
  xfsacih : Inport  Port=10
  w_xsdpan : Inport  Port=11
  xidld : Inport  Port=12
  xcol : Inport  Port=13
  xhpr_accut : Inport  Port=14
  xclcn : Inport  Port=15
  vspe : Inport  Port=16
  xstbymd_iss : Inport  Port=17
  xismd_iss : Inport  Port=18
  xirmd_iss : Inport  Port=19
  rgear : Inport  Port=20
  grade : Inport  Port=21
  xvspf : Inport  Port=22
  evatemp_uplmt : Inport  Port=23
  evatemp : Inport  Port=24
  iss_state : Inport  Port=25
  xclcncf : Inport  Port=26
  xacptc2f : Inport  Port=27
  vcv_cut_time : Inport  Port=28
  xnlidl : Inport  Port=29
  Constant3 : lib2011b/Simulink Original/Sources/MC_Constant  Value=0  datatype=uint16  SampleTime=inf  FramePeriod=inf  OutMin=[]  OutMax=[]  OutDataTypeStr=uint16
  MC_Constant : lib2011b/Simulink Original/Sources/MC_Constant  Value=false  datatype=Inherit: Inherit from 'Constant value'  SampleTime=inf  FramePeriod=inf  OutMin=[]  OutMax=[]  OutDataTypeStr=Inherit: Inherit from 'Constant value'
  MC_Constant1 : lib2011b/Simulink Original/Sources/MC_Constant  Value=true  datatype=Inherit: Inherit from 'Constant value'  SampleTime=inf  FramePeriod=inf  OutMin=[]  OutMax=[]  OutDataTypeStr=Inherit: Inherit from 'Constant value'
  MC_Constant2 : lib2011b/Simulink Original/Sources/MC_Constant  Value=false  datatype=Inherit: Inherit from 'Constant value'  SampleTime=inf  FramePeriod=inf  OutMin=[]  OutMax=[]  OutDataTypeStr=Inherit: Inherit from 'Constant value'
  MC_Constant3 : lib2011b/Simulink Original/Sources/MC_Constant  Value=false  datatype=Inherit: Inherit from 'Constant value'  SampleTime=inf  FramePeriod=inf  OutMin=[]  OutMax=[]  OutDataTypeStr=Inherit: Inherit from 'Constant value'
  MC_Constant4 : lib2011b/Simulink Original/Sources/MC_Constant  Value=KACC_EVATMPCUT_SW  datatype=Inherit: Inherit from 'Constant value'  SampleTime=inf  FramePeriod=inf  OutMin=[]  OutMax=[]  OutDataTypeStr=Inherit: Inherit from 'Constant value'
  MC_DataTypeConversion : lib2011b/Simulink Original/Signal Attributes/MC_DataTypeConversion  OutMin=[]  OutMax=[]  OutDataTypeStr=uint16  Signaltype=uint16  ConvertRealWorld=Real World Value (RWV)  RndMeth=Zero  SampleTime=-1
  MC_DataTypeConversion1 : lib2011b/Simulink Original/Signal Attributes/MC_DataTypeConversion  OutMin=[]  OutMax=[]  OutDataTypeStr=boolean  Signaltype=boolean  ConvertRealWorld=Real World Value (RWV)  RndMeth=Zero  SampleTime=-1
  MC_DownCountTimer : lib2011b/Mazda Library/Timer/MC_DownCountTimer
      settings: AttributesFormatString=DownCountTimer
  MC_Edge : SUBSYSTEM_LIB_CNV/RiseEdge
      settings: AttributesFormatString=RISE
  MC_Edge1 : SUBSYSTEM_LIB_CNV/RiseEdge
      settings: AttributesFormatString=RISE
  MC_LogicalOperator1 : lib2011b/Simulink Original/Logic and Bit Operations/MC_LogicalOperator  SelectedOperator=OR  Inputs=16  SampleTime=-1  AllPortsSameDT=off  OutDataTypeStr=boolean
  MC_LogicalOperator2 : lib2011b/Simulink Original/Logic and Bit Operations/MC_LogicalOperator  SelectedOperator=OR  Inputs=14  SampleTime=-1  AllPortsSameDT=off  OutDataTypeStr=boolean
  MC_LogicalOperator3 : lib2011b/Simulink Original/Logic and Bit Operations/MC_LogicalOperator  SelectedOperator=NOT  Inputs=2  SampleTime=-1  AllPortsSameDT=off  OutDataTypeStr=boolean
  MC_LogicalOperator4 : lib2011b/Simulink Original/Logic and Bit Operations/MC_LogicalOperator  SelectedOperator=AND  Inputs=2  SampleTime=-1  AllPortsSameDT=off  OutDataTypeStr=boolean
  MC_LogicalOperator6 : lib2011b/Simulink Original/Logic and Bit Operations/MC_LogicalOperator  SelectedOperator=OR  Inputs=2  SampleTime=-1  AllPortsSameDT=off  OutDataTypeStr=boolean
  MC_LogicalOperator7 : lib2011b/Simulink Original/Logic and Bit Operations/MC_LogicalOperator  SelectedOperator=OR  Inputs=2  SampleTime=-1  AllPortsSameDT=off  OutDataTypeStr=boolean
  MC_RelationalOperator : lib2011b/Simulink Original/Logic and Bit Operations/MC_RelationalOperator  Operator=>  SampleTime=-1  InputSameDT=on  OutDataTypeStr=boolean
  MC_UnitDelay2 : lib2011b/Simulink Original/Discrete/MC_UnitDelay  InitialCondition=0  InputProcessing=Inherited  SampleTime=-1  StateName=delay_yclcn_b20m9496
      settings: StateMustResolveToSignalObject=off  StateStorageClass=ExportedGlobal
  MC_UnitDelay3 : lib2011b/Simulink Original/Discrete/MC_UnitDelay  InitialCondition=0  InputProcessing=Inherited  SampleTime=-1  StateName=delay_yclcn_b20m9497
      settings: StateMustResolveToSignalObject=off  StateStorageClass=ExportedGlobal
  cal_cuttime : Subsystem
  do_xacct1 : Subsystem
      mask Display: disp('全開加速時A/Cカット')
  do_xacct4 : Subsystem
      mask Display: disp('発進時A/Cカット')
  do_xacflostcut : Subsystem
      mask Display: disp('フロスト限界ACカット')
  do_xacfrpm : Subsystem
      mask Display: disp('初回作動時の高回転A/Cカット')
  do_xacpcut : Subsystem
      mask Display: disp('冷媒圧条件A/Cカット')
  do_xactempcut : Subsystem
      mask Display: disp('エバ温条件A/COFF')
  do_xacuthil : Subsystem
      mask Display: disp('登坂時A/Cカット')
  do_xis_colof : Subsystem
      mask Display: disp('IS実行時A/Cカット')
  do_xlacfs : Subsystem
      mask Display: disp('始動時A/Cカット')
  do_xlacni : Subsystem
      mask Display: disp('高回転時A/Cカット')
  xaccuton : Outport
  xacct1 : Outport  Port=2
  xcolp : Outport  Port=3
  xemg_hldclr : Outport  Port=4
  xlacfs : Outport  Port=5
  xemg_accut : Outport  Port=6
  wires:
  xaltcalflg/1 -> [xaltcalflg]
  [ne] -> do_xacfrpm/1(ne)
  [apsfil] -> do_xacct1/2(apsfil)
  [xrload] -> do_xacct1/1(xrload)
  [ne] -> do_xlacni/1(ne)
  xbrst/1 -> [xbrst]
  apsfil/1 -> [apsfil]
  xrload/1 -> [xrload]
  gearp/1 -> [gearp]
  ne/1 -> [ne]
  xzst/1 -> [xzst]
  w_tsmpl/1 -> [w_tsmpl]
  xirmd_iss/1 -> [xirmd_iss]
  MC_Constant1/1 -> MC_DownCountTimer/3
  do_xlacfs/1(xlacfs) -> [xlacfs], xlacfs/1
  do_xlacni/1(xlacni) -> [xlacni]
  do_xacct1/1(xacct1) -> [xacct1]
  do_xacfrpm/1(xacfrpm) -> [xacfrpm]
  [xacct1] -> xacct1/1
  Constant3/1 -> MC_RelationalOperator/2
  do_xlacfs/2(xlacfs_iss) -> [xlacfs_iss]
  xidld/1 -> [xidld]
  xfsacih/1 -> [xfsacih]
  colp/1 -> [colp]
  w_xsdpan/1 -> [w_xsdpan]
  xcol/1 -> [xcol]
  MC_Constant/1 -> MC_Edge/2
  [xcol] -> MC_LogicalOperator3/1
  MC_Edge/1 -> MC_LogicalOperator6/1
  MC_LogicalOperator2/1 -> MC_Edge/1, MC_LogicalOperator7/1  "xaccut_wocnt"
  [w_tsmpl] -> do_xacpcut/2(w_tsmpl)
  [colp] -> do_xacpcut/1(colp)
  [xstbymd_iss] -> do_xis_colof/2(xstbymd_iss)
  [vspe] -> do_xis_colof/1(vspe)
  [xismd_iss] -> do_xis_colof/3(xismd_iss)
  [xirmd_iss] -> do_xis_colof/4(xirmd_iss)
  xismd_iss/1 -> [xismd_iss]
  xstbymd_iss/1 -> [xstbymd_iss]
  vspe/1 -> [vspe]
  xhpr_accut/1 -> [xhpr_accut]
  xclcn/1 -> MC_UnitDelay2/1
  [xcolp] -> xcolp/1
  do_xacpcut/2(xcolp) -> [xcolp]
  do_xis_colof/1(xis_colof) -> [xis_colof]
  do_xacpcut/1(xacpcut) -> [xacpcut]
  MC_RelationalOperator/1 -> MC_LogicalOperator7/2
  [xlacni] -> cal_cuttime/1(xlacni)
  [xlacfs] -> cal_cuttime/2(xlacfs)
  [xlacfs_iss] -> cal_cuttime/3(xlacfs_iss)
  MC_LogicalOperator7/1 -> xaccuton/1  "xaccuton"
  do_xacuthil/1(xacuthil) -> [xacuthil]
  [vspe] -> do_xacuthil/1(vspe)
  [apsfil] -> do_xacuthil/2(apsfil)
  [rgear] -> do_xacuthil/3(rgear)
  rgear/1 -> [rgear]
  MC_LogicalOperator6/1 -> MC_DownCountTimer/2
  [w_tsmpl] -> MC_DownCountTimer/5
  [xacfrpm] -> MC_LogicalOperator2/1
  [xfsacih] -> MC_LogicalOperator2/2
  [w_xsdpan] -> MC_LogicalOperator2/3
  [xis_colof] -> MC_LogicalOperator2/4
  [xacpcut] -> MC_LogicalOperator2/6
  MC_UnitDelay2/1 -> [xclcn]
  [xclcn] -> do_xacfrpm/2(xclcn)
  [xaltcalflg] -> do_xacfrpm/3(xaltcalflg)
  [w_tsmpl] -> do_xacuthil/5(w_tsmpl)
  [grade] -> do_xacuthil/4(grade)
  grade/1 -> [grade]
  [gearp] -> do_xacct1/3(gearp)
  [w_tsmpl] -> do_xacct1/4(w_tsmpl)
  MC_LogicalOperator3/1 -> MC_LogicalOperator2/7
  cal_cuttime/1(xaccut_wicnt) -> MC_LogicalOperator6/2
  do_xacct4/1(xacct4) -> [xacct4]
  [xrload] -> do_xacct4/1(xrload)
  [apsfil] -> do_xacct4/2(apsfil)
  [xidld] -> do_xacct4/3(xidld)
  [w_tsmpl] -> do_xacct4/6(w_tsmpl)
  [vspe] -> do_xacct4/4(vspe)
  [xvspf] -> do_xacct4/5(xvspf)
  xvspf/1 -> [xvspf]
  MC_LogicalOperator1/1 -> MC_Edge1/1, xemg_accut/1  "xemg_accut"
  MC_Constant3/1 -> MC_Edge1/2
  MC_Edge1/1 -> xemg_hldclr/1  "xemg_hldclr"
  [xacfrpm] -> MC_LogicalOperator1/1
  [xfsacih] -> MC_LogicalOperator1/2
  [w_xsdpan] -> MC_LogicalOperator1/3
  [xis_colof] -> MC_LogicalOperator1/4
  [xacpcut] -> MC_LogicalOperator1/5
  [xacuthil] -> MC_LogicalOperator1/6
  [xacct1] -> MC_LogicalOperator1/7
  [xacct4] -> MC_LogicalOperator1/8
  [xbrst] -> do_xlacfs/1(xbrst)
  [xzst] -> do_xlacfs/2(xzst)
  [xirmd_iss] -> do_xlacfs/3(xirmd_iss)
  cal_cuttime/2(accut_reqtime) -> MC_DownCountTimer/4
  MC_DownCountTimer/1 -> MC_DataTypeConversion/1
  MC_DataTypeConversion/1 -> MC_RelationalOperator/1  "caccuton"
  [xhpr_accut] -> MC_LogicalOperator2/5
  [xlacni] -> MC_LogicalOperator1/9
  [xlacfs] -> MC_LogicalOperator1/10
  [xlacfs_iss] -> MC_LogicalOperator1/11
  MC_Constant2/1 -> MC_DownCountTimer/1
  [xhpr_accut] -> MC_LogicalOperator1/12
  [xacuthil] -> MC_LogicalOperator2/8
  [xacct1] -> MC_LogicalOperator2/9
  [xacct4] -> MC_LogicalOperator2/10
  [evatemp_uplmt] -> do_xactempcut/1(evatemp_uplmt)
  [evatemp] -> do_xactempcut/2(evatemp)
  [apsfil] -> do_xactempcut/3(apsfil)
  do_xactempcut/1(xactempcut) -> [xactempcut]
  evatemp_uplmt/1 -> [evatemp_uplmt]
  evatemp/1 -> [evatemp]
  [xactempcut] -> MC_LogicalOperator2/11
  iss_state/1 -> do_xis_colof/5(iss_state)
  xclcncf/1 -> [xclcncf]
  [xclcncf] -> MC_LogicalOperator2/12
  xacptc2f/1 -> [xacptc2f]
  [xacptc2f] -> MC_LogicalOperator2/13
  [xcol] -> do_xacflostcut/1(xcol)
  [evatemp] -> do_xacflostcut/2(evatemp)
  do_xacflostcut/1(xacflostcut) -> [xacflostcut]
  [xacflostcut] -> MC_LogicalOperator2/14
  [xactempcut] -> MC_LogicalOperator4/1
  MC_Constant4/1 -> MC_DataTypeConversion1/1
  [xclcncf] -> MC_LogicalOperator1/13
  [xacptc2f] -> MC_LogicalOperator1/14
  [xacflostcut] -> MC_LogicalOperator1/15
  MC_LogicalOperator4/1 -> MC_LogicalOperator1/16
  MC_DataTypeConversion1/1 -> MC_LogicalOperator4/2
  vcv_cut_time/1 -> MC_UnitDelay3/1
  MC_UnitDelay3/1 -> [w_vcv_cut_time]
  [w_vcv_cut_time] -> cal_cuttime/4(w_vcv_cut_time)
  [xacct1] -> cal_cuttime/5(xacct1)
  [xacct4] -> cal_cuttime/6(xacct4)
  [xacuthil] -> cal_cuttime/7(xacuthil)
  [xactempcut] -> cal_cuttime/8(xactempcut)
  [xnlidl] -> do_xacct4/7(xnlidl)
  xnlidl/1 -> [xnlidl]

== system filecuaho/acc_xyclcn/set_init1 ==
  note: /* トルクベース制御 エアコンOFFディレー */
  note: ↑/* 可変容量A/Cユニーク エアコンOFFディレー(TPV検証用)*/
  note: /* トルクベース制御 エアコンOFFディレー */
  ne : Inport
  xrload : Inport  Port=2
  tqe_rsv_ac : Inport  Port=3
  Enable : EnablePort
  Constant1 : lib2011b/Simulink Original/Sources/MC_Constant  Value=KACC_OFDL_VCV  datatype=Inherit: Inherit from 'Constant value'  SampleTime=inf  FramePeriod=inf  OutMin=[]  OutMax=[]  OutDataTypeStr=Inherit: Inherit from 'Constant value'
  Constant2 : lib2011b/Simulink Original/Sources/MC_Constant  Value=KACC_OFDL_SW  datatype=Inherit: Inherit from 'Constant value'  SampleTime=inf  FramePeriod=inf  OutMin=[]  OutMax=[]  OutDataTypeStr=Inherit: Inherit from 'Constant value'
  MC_DataTypeConversion : lib2011b/Simulink Original/Signal Attributes/MC_DataTypeConversion  OutMin=[]  OutMax=[]  OutDataTypeStr=boolean  Signaltype=boolean  ConvertRealWorld=Real World Value (RWV)  RndMeth=Zero  SaturateOnIntegerOverflow=on  SampleTime=-1
  MC_Map_i : lib2011b/Simulink Original/Lookup Tables/MC_Map_i  Label=MACC_OFDLY_TQMR  ColumnIndex=TACC_OFDLY_TQMR_X  calsw_x=on  RowIndex=TACC_OFDLY_TQMR_Y  calsw_y=on  OutputValues=MACC_OFDLY_TQMR_Z  LsbValue=LSB_MACC_OFDLY_TQMR_Z  OffsetValue=OFFSET_MACC_OFDLY_TQMR_Z
      settings: AttributesFormatString=%<Label>\nX-axis %<calsw_x>, Y-axis %<calsw_y>
  MC_Map_i1 : lib2011b/Simulink Original/Lookup Tables/MC_Map_i  Label=MACC_OFDLY_TQMN  ColumnIndex=TACC_OFDLY_TQMN_X  calsw_x=on  RowIndex=TACC_OFDLY_TQMN_Y  calsw_y=on  OutputValues=MACC_OFDLY_TQMN_Z  LsbValue=LSB_MACC_OFDLY_TQMN_Z  OffsetValue=OFFSET_MACC_OFDLY_TQMN_Z
      settings: AttributesFormatString=%<Label>\nX-axis %<calsw_x>, Y-axis %<calsw_y>
  MC_MinMax1 : lib2011b/Simulink Original/Math Operations/MC_MinMax  Function=max  Inputs=2  SampleTime=-1  InputSameDT=on  OutMin=[]  OutMax=[]
  Switch1 : lib2011b/Simulink Original/Signal Routing/MC_Switch  Criteria=u2 ~= 0  Threshold=0  SampleTime=-1  InputSameDT=on  OutMin=[]  OutMax=[]  AllowDiffInputSizes=off
  Switch2 : lib2011b/Simulink Original/Signal Routing/MC_Switch  Criteria=u2 ~= 0  Threshold=0  SampleTime=-1  InputSameDT=on  OutMin=[]  OutMax=[]  AllowDiffInputSizes=off
  Switch3 : lib2011b/Simulink Original/Signal Routing/MC_Switch  Criteria=u2 ~= 0  Threshold=0  SampleTime=-1  InputSameDT=on  OutMin=[]  OutMax=[]  AllowDiffInputSizes=off
  TLACDFN1 : lib2011b/Simulink Original/Lookup Tables/MC_Table_i  Label=TACC_OFDL_TQMR  InputValues=TACC_OFDL_TQMR_X  calsw_x=off  OutputValues=TACC_OFDL_TQMR_Y  LsbValue=LSB_TACC_OFDL_TQMR_Y  OffsetValue=OFFSET_TACC_OFDL_TQMR_Y
      settings: AttributesFormatString=%<Label>\nX-axis %<calsw_x>
  TLACDFN2 : lib2011b/Simulink Original/Lookup Tables/MC_Table_i  Label=TACC_OFDL_TQMN  InputValues=TACC_OFDL_TQMN_X  calsw_x=off  OutputValues=TACC_OFDL_TQMN_Y  LsbValue=LSB_TACC_OFDL_TQMN_Y  OffsetValue=OFFSET_TACC_OFDL_TQMN_Y
      settings: AttributesFormatString=%<Label>\nX-axis %<calsw_x>
  w_init : Outport
  wires:
  xrload/1 -> [xrload]
  [xrload] -> Switch3/2
  ne/1 -> [ne]
  TLACDFN1/1 -> Switch3/1
  TLACDFN2/1 -> Switch3/3
  [ne] -> TLACDFN1/1
  [ne] -> TLACDFN2/1
  MC_MinMax1/1 -> w_init/1  "w_init"
  Constant1/1 -> MC_MinMax1/2
  Switch1/1 -> Switch2/1
  Constant2/1 -> MC_DataTypeConversion/1
  MC_DataTypeConversion/1 -> Switch2/2
  tqe_rsv_ac/1 -> [tqe_rsv_ac]
  MC_Map_i/1 -> Switch1/1
  MC_Map_i1/1 -> Switch1/3
  [tqe_rsv_ac] -> MC_Map_i/1
  [ne] -> MC_Map_i/2
  [tqe_rsv_ac] -> MC_Map_i1/1
  [ne] -> MC_Map_i1/2
  [xrload] -> Switch1/2
  Switch3/1 -> Switch2/3
  Switch2/1 -> MC_MinMax1/1

== system filecuaho/acc_xyclcn/set_init2 ==
  note: /* トルクベース制御 エアコンONディレー */
  note: /* トルクベース制御 エアコンONディレー */
  ne : Inport
  xrload : Inport  Port=2
  tqe_rsv_ac : Inport  Port=3
  Enable : EnablePort
  Constant2 : lib2011b/Simulink Original/Sources/MC_Constant  Value=KACC_ONDL_SW  datatype=Inherit: Inherit from 'Constant value'  SampleTime=inf  FramePeriod=inf  OutMin=[]  OutMax=[]  OutDataTypeStr=Inherit: Inherit from 'Constant value'
  MC_DataTypeConversion : lib2011b/Simulink Original/Signal Attributes/MC_DataTypeConversion  OutMin=[]  OutMax=[]  OutDataTypeStr=boolean  Signaltype=boolean  ConvertRealWorld=Real World Value (RWV)  RndMeth=Zero  SaturateOnIntegerOverflow=on  SampleTime=-1
  MC_Map_i : lib2011b/Simulink Original/Lookup Tables/MC_Map_i  Label=MACC_ONDLY_TQMR  ColumnIndex=TACC_ONDLY_TQMR_X  calsw_x=on  RowIndex=TACC_ONDLY_TQMR_Y  calsw_y=on  OutputValues=MACC_ONDLY_TQMR_Z  LsbValue=LSB_MACC_ONDLY_TQMR_Z  OffsetValue=OFFSET_MACC_ONDLY_TQMR_Z
      settings: AttributesFormatString=%<Label>\nX-axis %<calsw_x>, Y-axis %<calsw_y>
  MC_Map_i1 : lib2011b/Simulink Original/Lookup Tables/MC_Map_i  Label=MACC_ONDLY_TQMN  ColumnIndex=TACC_ONDLY_TQMN_X  calsw_x=on  RowIndex=TACC_ONDLY_TQMN_Y  calsw_y=on  OutputValues=MACC_ONDLY_TQMN_Z  LsbValue=LSB_MACC_ONDLY_TQMN_Z  OffsetValue=OFFSET_MACC_ONDLY_TQMN_Z
      settings: AttributesFormatString=%<Label>\nX-axis %<calsw_x>, Y-axis %<calsw_y>
  Switch1 : lib2011b/Simulink Original/Signal Routing/MC_Switch  Criteria=u2 ~= 0  Threshold=0  SampleTime=-1  InputSameDT=on  OutMin=[]  OutMax=[]  AllowDiffInputSizes=off
  Switch2 : lib2011b/Simulink Original/Signal Routing/MC_Switch  Criteria=u2 ~= 0  Threshold=0  SampleTime=-1  InputSameDT=on  OutMin=[]  OutMax=[]  AllowDiffInputSizes=off
  Switch6 : lib2011b/Simulink Original/Signal Routing/MC_Switch  Criteria=u2 ~= 0  Threshold=0  SampleTime=-1  InputSameDT=on  OutMin=[]  OutMax=[]  AllowDiffInputSizes=off
  TLACDFN1 : lib2011b/Simulink Original/Lookup Tables/MC_Table_i  Label=TACC_ONDL_TQMR  InputValues=TACC_ONDL_TQMR_X  calsw_x=off  OutputValues=TACC_ONDL_TQMR_Y  LsbValue=LSB_TACC_ONDL_TQMR_Y  OffsetValue=OFFSET_TACC_ONDL_TQMR_Y
      settings: AttributesFormatString=%<Label>\nX-axis %<calsw_x>
  TLACDFN2 : lib2011b/Simulink Original/Lookup Tables/MC_Table_i  Label=TACC_ONDL_TQMN  InputValues=TACC_ONDL_TQMN_X  calsw_x=off  OutputValues=TACC_ONDL_TQMN_Y  LsbValue=LSB_TACC_ONDL_TQMN_Y  OffsetValue=OFFSET_TACC_ONDL_TQMN_Y
      settings: AttributesFormatString=%<Label>\nX-axis %<calsw_x>
  w_init : Outport
  wires:
  [ne] -> TLACDFN1/1
  [ne] -> TLACDFN2/1
  TLACDFN1/1 -> Switch6/1
  [xrload] -> Switch6/2
  TLACDFN2/1 -> Switch6/3
  ne/1 -> [ne]
  xrload/1 -> [xrload]
  [xrload] -> Switch1/2
  Switch1/1 -> Switch2/1
  Constant2/1 -> MC_DataTypeConversion/1
  MC_DataTypeConversion/1 -> Switch2/2
  MC_Map_i/1 -> Switch1/1
  MC_Map_i1/1 -> Switch1/3
  tqe_rsv_ac/1 -> [tqe_rsv_ac]
  [tqe_rsv_ac] -> MC_Map_i/1
  [ne] -> MC_Map_i/2
  [tqe_rsv_ac] -> MC_Map_i1/1
  [ne] -> MC_Map_i1/2
  Switch6/1 -> Switch2/3
  Switch2/1 -> w_init/1  "w_init"
